simulink model "cantp"  (R2020a)
settings: Solver=VariableStepAuto  StartTime=0.0  StopTime=inf  RelTol=1e-3
InitFcn:
  | messagePeriod=1.0;%must be greater than 5ms.
  | 
  | Fsquare=1;
  | squareTs=0.01/Fsquare;
  | squareSamplesPerPeriod=fix(1/Fsquare/squareTs);
  | squareSamplesPerPulseWidth=fix(squareSamplesPerPeriod/2);
  | squareAmplitude=1;
  | 
  | Fsinus=0.05;
  | sinusTs=0.01/Fsinus;
  | sinusSamplesPerPeriod=fix(1/Fsinus/sinusTs);
  | sinusAmplitude=100;
  | rxCANSampleTime=0.01;
undefined symbols (not defined in the file): canChannel
libraries: canlib x14, canmsglib x14, simulink x6
(part 1 of 2)
settings Model: Creator=pc  LastModifiedBy=HP
settings DataIOCC: ReturnWorkspaceOutputs=off
settings DebuggingCC: ArithmeticOperatorsInVariantConditions=warning
settings SFSimCC: SimUseLocalCustomCode=off  CustomCodeUndefinedFunction=UseInterfaceOnly
settings RTWCC: RTWUseLocalCustomCode=off

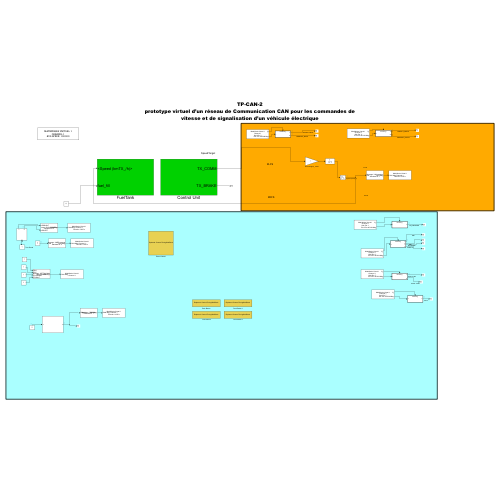
[thumbnail: Simulink's stored preview of the top-level diagram]
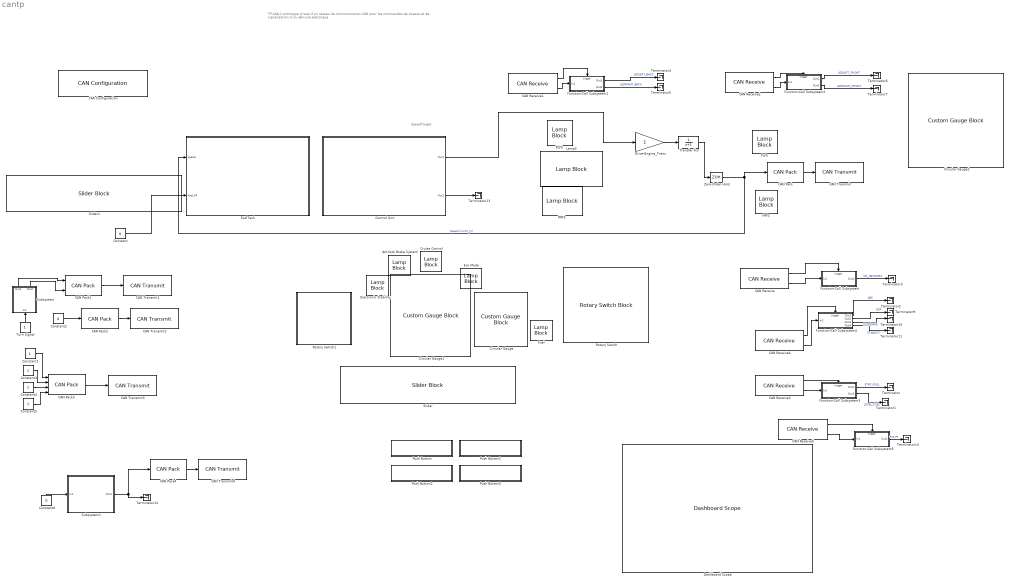
== system cantp ==
  note: SpeedTarget
  note: TP-CAN-2
      | prototype virtuel d’un réseau de Communication CAN pour les commandes de vitesse et de signalisation d’un véhicule électrique
  Antilock Brake System : LampBlock  LabelPosition=Hide  Icon=AntilockBrakeSystem
  CAN Configuration : canlib/CAN Configuration  BlockHandle=303.0002  Device=MathWorks Virtual 1 (Channel 1)  DeviceMenu=MathWorks Virtual 1 (Channel 1)  ObjConstructor=canChannel('MathWorks', 'Virtual 1', 1)  BusSpeed=100000  EnableBitParameters=off  AckMode=Normal
      settings: SourceProductBaseCode=VN
  CAN Pack : canmsglib/CAN Pack  MsgList=(none)  MsgName=VM message  MsgIDType=Standard (11-bit identifier)  MsgIdentifier=1  MsgLength=4  Remote=off  ApplyMinMax=off  BusOutput=off  SignalInfo={ 'VW', '0', '8', 'LE', 'unsigned', 'Standard', '0', '1', '0', '-Inf', 'Inf' }
      settings: SourceProductBaseCode=ME,XP,VN  DataFormat=manually specified signals
  CAN Pack1 : canmsglib/CAN Pack  MsgList=(none)  MsgName=DASHBOARD msg  MsgIDType=Standard (11-bit identifier)  MsgIdentifier=2  MsgLength=1  Remote=off  ApplyMinMax=off  BusOutput=off  SignalInfo={ 'LEDRIGHT', '0', '1', 'LE', 'unsigned', 'Standard', '0', '1', '0', '0', '1'; 'LEDLEFT', '1', '1', 'LE', 'unsigned', 'Standard', '0', '1', '0', '0', '1' }
      settings: SourceProductBaseCode=ME,XP,VN  DataFormat=manually specified signals
  CAN Pack2 : canmsglib/CAN Pack  MsgList=(none)  MsgName=VMES message  MsgIDType=Standard (11-bit identifier)  MsgIdentifier=3  MsgLength=2  Remote=off  ApplyMinMax=off  BusOutput=off  SignalInfo={ 'VM', '0', '8', 'LE', 'unsigned', 'Standard', '0', '1', '0', '0', '255' }
      settings: SourceProductBaseCode=ME,XP,VN  DataFormat=manually specified signals
  CAN Pack3 : canmsglib/CAN Pack  MsgList=(none)  MsgName=SETTING Msg  MsgIDType=Standard (11-bit identifier)  MsgIdentifier=6  MsgLength=1  Remote=off  ApplyMinMax=off  BusOutput=off  SignalInfo={ 'ABS', '0', '1', 'LE', 'unsigned', 'Standard', '0', '1', '0', '0', '1'; 'ESP', '1', '1', 'LE', 'unsigned', 'Standard', '0', '1', '0', '0', '1'; 'ECONOMIC', '2', '1', 'LE', 'unsigned', 'Standard', '0', '1', '0', '0', '1'; 'STABILIT', '3', '1', 'LE', 'unsigned', 'Standard', '0', '1', '0', '0', '1' }
      settings: SourceProductBaseCode=ME,XP,VN  DataFormat=manually specified signals
  CAN Pack4 : canmsglib/CAN Pack  MsgList=(none)  MsgName=CAN Msg  MsgIDType=Standard (11-bit identifier)  MsgIdentifier=7  MsgLength=1  Remote=off  ApplyMinMax=off  BusOutput=off  SignalInfo={ 'Signal1', '0', '1', 'LE', 'unsigned', 'Standard', '0', '1', '0', '0', '1' }
      settings: SourceProductBaseCode=ME,XP,VN  DataFormat=manually specified signals
  CAN Receive : canlib/CAN Receive  BlockHandle=309.0002  Device=MathWorks Virtual 1 (Channel 1)  DeviceMenu=MathWorks Virtual 1 (Channel 1)  ObjConstructor=canChannel('MathWorks', 'Virtual 1', 1)  EnableStandardIDsFilter=off  StdIDsCombo=Allow only  StandardIDs=1  EnableExtendedIDsFilter=off  ExtIDsCombo=Allow all  ExtendedIDs=0  SampleTime=0.01  MsgsPerTimestep=all  InternalFilterUpdateStatus=on  BusOutput=off
      settings: SourceProductBaseCode=VN
  CAN Receive1 : canlib/CAN Receive  BlockHandle=310.0002  Device=MathWorks Virtual 1 (Channel 1)  DeviceMenu=MathWorks Virtual 1 (Channel 1)  ObjConstructor=canChannel('MathWorks', 'Virtual 1', 1)  EnableStandardIDsFilter=off  StdIDsCombo=Allow only  StandardIDs=2  EnableExtendedIDsFilter=off  ExtIDsCombo=Allow all  ExtendedIDs=0  SampleTime=0.01  MsgsPerTimestep=all  InternalFilterUpdateStatus=on  BusOutput=off
      settings: SourceProductBaseCode=VN
  CAN Receive2 : canlib/CAN Receive  BlockHandle=528.0004  Device=MathWorks Virtual 1 (Channel 1)  DeviceMenu=MathWorks Virtual 1 (Channel 1)  ObjConstructor=canChannel('MathWorks', 'Virtual 1', 1)  EnableStandardIDsFilter=off  StdIDsCombo=Allow only  StandardIDs=2  EnableExtendedIDsFilter=off  ExtIDsCombo=Allow all  ExtendedIDs=0  SampleTime=0.01  MsgsPerTimestep=all  InternalFilterUpdateStatus=on  BusOutput=off
      settings: SourceProductBaseCode=VN
  CAN Receive3 : canlib/CAN Receive  BlockHandle=529.0004  Device=MathWorks Virtual 1 (Channel 1)  DeviceMenu=MathWorks Virtual 1 (Channel 1)  ObjConstructor=canChannel('MathWorks', 'Virtual 1', 1)  EnableStandardIDsFilter=off  StdIDsCombo=Allow only  StandardIDs=5  EnableExtendedIDsFilter=off  ExtIDsCombo=Allow all  ExtendedIDs=0  SampleTime=0.01  MsgsPerTimestep=all  InternalFilterUpdateStatus=on  BusOutput=off
      settings: SourceProductBaseCode=VN
  CAN Receive4 : canlib/CAN Receive  BlockHandle=530.0004  Device=MathWorks Virtual 1 (Channel 1)  DeviceMenu=MathWorks Virtual 1 (Channel 1)  ObjConstructor=canChannel('MathWorks', 'Virtual 1', 1)  EnableStandardIDsFilter=off  StdIDsCombo=Allow only  StandardIDs=6  EnableExtendedIDsFilter=off  ExtIDsCombo=Allow all  ExtendedIDs=0  SampleTime=0.01  MsgsPerTimestep=all  InternalFilterUpdateStatus=on  BusOutput=off
      settings: SourceProductBaseCode=VN
  CAN Receive5 : canlib/CAN Receive  BlockHandle=531.0002  Device=MathWorks Virtual 1 (Channel 1)  DeviceMenu=MathWorks Virtual 1 (Channel 1)  ObjConstructor=canChannel('MathWorks', 'Virtual 1', 1)  EnableStandardIDsFilter=off  StdIDsCombo=Allow only  StandardIDs=7  EnableExtendedIDsFilter=off  ExtIDsCombo=Allow all  ExtendedIDs=0  SampleTime=0.01  MsgsPerTimestep=all  InternalFilterUpdateStatus=on  BusOutput=off
      settings: SourceProductBaseCode=VN
  CAN Transmit : canlib/CAN Transmit  BlockHandle=532.0002  Device=MathWorks Virtual 1 (Channel 1)  DeviceMenu=MathWorks Virtual 1 (Channel 1)  ObjConstructor=canChannel('MathWorks', 'Virtual 1', 1)  EnableEventTransmit=off  EnablePeriodicTransmit=on  MessagePeriod=0.025
      settings: SourceProductBaseCode=VN
  CAN Transmit1 : canlib/CAN Transmit  BlockHandle=533.0002  Device=MathWorks Virtual 1 (Channel 1)  DeviceMenu=MathWorks Virtual 1 (Channel 1)  ObjConstructor=canChannel('MathWorks', 'Virtual 1', 1)  EnableEventTransmit=off  EnablePeriodicTransmit=on  MessagePeriod=0.025
      settings: SourceProductBaseCode=VN
  CAN Transmit2 : canlib/CAN Transmit  BlockHandle=534.0002  Device=MathWorks Virtual 1 (Channel 1)  DeviceMenu=MathWorks Virtual 1 (Channel 1)  ObjConstructor=canChannel('MathWorks', 'Virtual 1', 1)  EnableEventTransmit=off  EnablePeriodicTransmit=on  MessagePeriod=0.025
      settings: SourceProductBaseCode=VN
  CAN Transmit3 : canlib/CAN Transmit  BlockHandle=535.0002  Device=MathWorks Virtual 1 (Channel 1)  DeviceMenu=MathWorks Virtual 1 (Channel 1)  ObjConstructor=canChannel('MathWorks', 'Virtual 1', 1)  EnableEventTransmit=off  EnablePeriodicTransmit=off  MessagePeriod=1.000
      settings: SourceProductBaseCode=VN
  CAN Transmit4 : canlib/CAN Transmit  BlockHandle=536.0002  Device=MathWorks Virtual 1 (Channel 1)  DeviceMenu=MathWorks Virtual 1 (Channel 1)  ObjConstructor=canChannel('MathWorks', 'Virtual 1', 1)  EnableEventTransmit=off  EnablePeriodicTransmit=on  MessagePeriod=0.025
      settings: SourceProductBaseCode=VN
  Circular Gauge : CustomGaugeBlock  LabelPosition=Hide  ShowInitialText=on  LabelPosition=Hide  ScaleMin=0  ScaleMax=100  TickInterval=auto  fixedAspectRatio=on  GaugeMin=0  GaugeMax=100  GaugeArcDefined=true  GaugeArcRadius=0.18125  GaugeArcStrokeWidth=0.03295454545454546  GaugeArcColor=#fcfcc5  GaugeArcRotation=225  GaugeArcRatio=0.75  GaugeArcTransparency=0  ValueArcTransparency=1  ValueArcColor=#0072bd  GaugeTickVisible=1  GaugeTickTransparency=1  GaugeTickColor=#fcfcc5  ScaleColorsJSON=[]  CenterOffsetX=-0.00375  CenterOffsetY=-0.00515625  NeedleImage=data:image/svg+xml;base64,PD94bWwgdmVyc2lvbj0iMS4wIiBlbmNvZGluZz0idXRmLTgiPz4KPCEtLSBHZW5lcmF0b3I6IEFkb2JlIElsbHVzdHJhdG9yIDI0LjEuMiwgU1ZHIEV4cG9ydCBQbHVnLUluIC4gU1ZHIFZlcnNpb246IDYuMDAgQnVpbGQgMCkgIC0tPgo8c3ZnIHZlcnNpb249IjEuMSIgaWQ9IkxheWVyXzEiIHhtbG5zPSJodHRwOi8vd3d3LnczLm9yZy8yMDAwL3N2ZyIgeG1sbnM6eGxpbms9Imh0dHA6Ly93d3cudzMub3JnLzE5OTkveGxpbmsiIHg9IjBweCIgeT0iMHB4IgoJIHZpZXdCb3g9IjAgMCAyMDAgNTAiIHN0eWxlPSJlbmFibGUtYmFja2dyb3VuZDpuZXcgMCAwIDIwMCA1MDsiIHhtbDpzcGFjZT0icHJlc2VydmUiPgo8c3R5bGUgdHlwZT0idGV4dC9jc3MiPgoJLnN0MHtmaWxsOiNFQzIxMjc7fQo8L3N0eWxlPgo8cGF0aCBjbGFzcz0ic3QwIiBkPSJNMTYyLjgsMTMuN0MxNjksNC40LDE4MS43LDEuOSwxOTEsOC4xczExLjgsMTguOSw1LjYsMjguMnMtMTguOSwxMS44LTI4LjIsNS42bDAsMAoJQzE1OS4xLDM1LjYsMTU2LjYsMjMsMTYyLjgsMTMuN0wxNjIuOCwxMy43eiBNMTY1LjgsMTUuOGMtNS4xLDcuNi0zLjEsMTcuOSw0LjYsMjNjNy42LDUuMSwxNy45LDMuMSwyMy00LjYKCWM1LjEtNy42LDMuMS0xNy45LTQuNi0yM2wwLDBDMTgxLjIsNi4yLDE3MC45LDguMiwxNjUuOCwxNS44eiIvPgo8cGF0aCBjbGFzcz0ic3QwIiBkPSJNMC40LDI1Ljl2LTMuM2wxNTktMi41Yy0wLjcsMi42LTAuNyw1LjIsMCw3LjhMMC40LDI1Ljl6Ii8+CjxjaXJjbGUgY2xhc3M9InN0MCIgY3g9IjE3OS42IiBjeT0iMjQiIHI9IjAuNyIvPgo8L3N2Zz4K  NeedleXPos=0.3459906005859375  NeedleYPos=0.5370294189453125  NeedleHeight=0.05870846152673457  NeedleWidth=0.23054168772545627  NeedleInitialRotation=-45  BackgroundImage=data:image/svg+xml;base64,PD94bWwgdmVyc2lvbj0iMS4wIiBlbmNvZGluZz0iVVRGLTgiIHN0YW5kYWxvbmU9Im5vIj8+CjxzdmcKICAgeG1sbnM6ZGM9Imh0dHA6Ly9wdXJsLm9yZy9kYy9lbGVtZW50cy8xLjEvIgogICB4bWxuczpjYz0iaHR0cDovL2NyZWF0aXZlY29tbW9ucy5vcmcvbnMjIgogICB4bWxuczpyZGY9Imh0dHA6Ly93d3cudzMub3JnLzE5OTkvMDIvMjItcmRmLXN5bnRheC1ucyMiCiAgIHhtbG5zOnN2Zz0iaHR0cDovL3d3dy53My5vcmcvMjAwMC9zdmciCiAgIHhtbG5zPSJodHRwOi8vd3d3LnczLm9yZy8yMDAwL3N2ZyIKICAgeG1sbnM6 ...(+9964 chars)
  Circular Gauge1 : CustomGaugeBlock  LabelPosition=Hide  ShowInitialText=on  LabelPosition=Hide  ScaleMin=0  ScaleMax=240  TickInterval=auto  fixedAspectRatio=on  GaugeMin=0  GaugeMax=240  GaugeArcDefined=true  GaugeArcRadius=0.18032212885154061  GaugeArcStrokeWidth=0.03278584160937103  GaugeArcColor=#fcfcc5  GaugeArcRotation=225  GaugeArcRatio=0.75  GaugeArcTransparency=0  ValueArcTransparency=1  ValueArcColor=#0072bd  GaugeTickVisible=1  GaugeTickTransparency=1  GaugeTickColor=#fcfcc5  ScaleColorsJSON=[]  CenterOffsetX=-0.00375  CenterOffsetY=0.0027573529411764708  NeedleImage=data:image/svg+xml;base64,PD94bWwgdmVyc2lvbj0iMS4wIiBlbmNvZGluZz0idXRmLTgiPz4KPCEtLSBHZW5lcmF0b3I6IEFkb2JlIElsbHVzdHJhdG9yIDI0LjEuMiwgU1ZHIEV4cG9ydCBQbHVnLUluIC4gU1ZHIFZlcnNpb246IDYuMDAgQnVpbGQgMCkgIC0tPgo8c3ZnIHZlcnNpb249IjEuMSIgaWQ9IkxheWVyXzEiIHhtbG5zPSJodHRwOi8vd3d3LnczLm9yZy8yMDAwL3N2ZyIgeG1sbnM6eGxpbms9Imh0dHA6Ly93d3cudzMub3JnLzE5OTkveGxpbmsiIHg9IjBweCIgeT0iMHB4IgoJIHZpZXdCb3g9IjAgMCAyMDAgNTAiIHN0eWxlPSJlbmFibGUtYmFja2dyb3VuZDpuZXcgMCAwIDIwMCA1MDsiIHhtbDpzcGFjZT0icHJlc2VydmUiPgo8c3R5bGUgdHlwZT0idGV4dC9jc3MiPgoJLnN0MHtmaWxsOiNFQzIxMjc7fQo8L3N0eWxlPgo8cGF0aCBjbGFzcz0ic3QwIiBkPSJNMTYyLjgsMTMuN0MxNjksNC40LDE4MS43LDEuOSwxOTEsOC4xczExLjgsMTguOSw1LjYsMjguMnMtMTguOSwxMS44LTI4LjIsNS42bDAsMAoJQzE1OS4xLDM1LjYsMTU2LjYsMjMsMTYyLjgsMTMuN0wxNjIuOCwxMy43eiBNMTY1LjgsMTUuOGMtNS4xLDcuNi0zLjEsMTcuOSw0LjYsMjNjNy42LDUuMSwxNy45LDMuMSwyMy00LjYKCWM1LjEtNy42LDMuMS0xNy45LTQuNi0yM2wwLDBDMTgxLjIsNi4yLDE3MC45LDguMiwxNjUuOCwxNS44eiIvPgo8cGF0aCBjbGFzcz0ic3QwIiBkPSJNMC40LDI1Ljl2LTMuM2wxNTktMi41Yy0wLjcsMi42LTAuNyw1LjIsMCw3LjhMMC40LDI1Ljl6Ii8+CjxjaXJjbGUgY2xhc3M9InN0MCIgY3g9IjE3OS42IiBjeT0iMjQiIHI9IjAuNyIvPgo8L3N2Zz4K  NeedleXPos=0.34361348470052083  NeedleYPos=0.5332382301879085  NeedleHeight=0.05870846152673456  NeedleWidth=0.2260212624759375  NeedleInitialRotation=-45  BackgroundImage=data:image/svg+xml;base64,PD94bWwgdmVyc2lvbj0iMS4wIiBlbmNvZGluZz0iVVRGLTgiIHN0YW5kYWxvbmU9Im5vIj8+CjxzdmcKICAgeG1sbnM6ZGM9Imh0dHA6Ly9wdXJsLm9yZy9kYy9lbGVtZW50cy8xLjEvIgogICB4bWxuczpjYz0iaHR0cDovL2NyZWF0aXZlY29tbW9ucy5vcmcvbnMjIgogICB4bWxuczpyZGY9Imh0dHA6Ly93d3cudzMub3JnLzE5OTkvMDIvMjItcmRmLXN5bnRheC1ucyMiCiAgIHhtbG5zOnN2Zz0iaHR0cDovL3d3dy53My5vcmcvMjAwMC9zdmciCiAgIHhtbG5zPSJodHRwOi8vd3d3LnczLm9yZy8yMDAwL3N2ZyIKICAgeG1sbnM6 ...(+9964 chars)
  Circular Gauge2 : CustomGaugeBlock  LabelPosition=Hide  ShowInitialText=on  LabelPosition=Hide  ScaleMin=0  ScaleMax=1  TickInterval=auto  fixedAspectRatio=on  GaugeMin=0  GaugeMax=1  GaugeArcDefined=true  GaugeArcRadius=0.1781875438904494  GaugeArcStrokeWidth=0.03239773525280899  GaugeArcColor=#fcfcc5  GaugeArcRotation=225  GaugeArcRatio=0.75  GaugeArcTransparency=0  ValueArcTransparency=0  ValueArcColor=#0072bd  GaugeTickVisible=1  GaugeTickTransparency=0  GaugeTickColor=#fcfcc5  ScaleColorsJSON=[]  CenterOffsetX=0.00008778089887640449  CenterOffsetY=-0.0009821428571428572  NeedleImage=data:image/svg+xml;base64,PD94bWwgdmVyc2lvbj0iMS4wIiBlbmNvZGluZz0idXRmLTgiPz4KPCEtLSBHZW5lcmF0b3I6IEFkb2JlIElsbHVzdHJhdG9yIDI0LjEuMiwgU1ZHIEV4cG9ydCBQbHVnLUluIC4gU1ZHIFZlcnNpb246IDYuMDAgQnVpbGQgMCkgIC0tPgo8c3ZnIHZlcnNpb249IjEuMSIgaWQ9IkxheWVyXzEiIHhtbG5zPSJodHRwOi8vd3d3LnczLm9yZy8yMDAwL3N2ZyIgeG1sbnM6eGxpbms9Imh0dHA6Ly93d3cudzMub3JnLzE5OTkveGxpbmsiIHg9IjBweCIgeT0iMHB4IgoJIHZpZXdCb3g9IjAgMCAyMDAgNTAiIHN0eWxlPSJlbmFibGUtYmFja2dyb3VuZDpuZXcgMCAwIDIwMCA1MDsiIHhtbDpzcGFjZT0icHJlc2VydmUiPgo8c3R5bGUgdHlwZT0idGV4dC9jc3MiPgoJLnN0MHtmaWxsOiNFQzIxMjc7fQo8L3N0eWxlPgo8cGF0aCBjbGFzcz0ic3QwIiBkPSJNMTYyLjgsMTMuN0MxNjksNC40LDE4MS43LDEuOSwxOTEsOC4xczExLjgsMTguOSw1LjYsMjguMnMtMTguOSwxMS44LTI4LjIsNS42bDAsMAoJQzE1OS4xLDM1LjYsMTU2LjYsMjMsMTYyLjgsMTMuN0wxNjIuOCwxMy43eiBNMTY1LjgsMTUuOGMtNS4xLDcuNi0zLjEsMTcuOSw0LjYsMjNjNy42LDUuMSwxNy45LDMuMSwyMy00LjYKCWM1LjEtNy42LDMuMS0xNy45LTQuNi0yM2wwLDBDMTgxLjIsNi4yLDE3MC45LDguMiwxNjUuOCwxNS44eiIvPgo8cGF0aCBjbGFzcz0ic3QwIiBkPSJNMC40LDI1Ljl2LTMuM2wxNTktMi41Yy0wLjcsMi42LTAuNyw1LjIsMCw3LjhMMC40LDI1Ljl6Ii8+CjxjaXJjbGUgY2xhc3M9InN0MCIgY3g9IjE3OS42IiBjeT0iMjQiIHI9IjAuNyIvPgo8L3N2Zz4K  NeedleXPos=0.45904198121488765  NeedleYPos=0.5336383492606026  NeedleHeight=0.0577189930740368  NeedleWidth=0.23054168772545627  NeedleInitialRotation=-45  BackgroundImage=data:image/svg+xml;base64,PD94bWwgdmVyc2lvbj0iMS4wIiBlbmNvZGluZz0iVVRGLTgiIHN0YW5kYWxvbmU9Im5vIj8+CjxzdmcKICAgeG1sbnM6ZGM9Imh0dHA6Ly9wdXJsLm9yZy9kYy9lbGVtZW50cy8xLjEvIgogICB4bWxuczpjYz0iaHR0cDovL2NyZWF0aXZlY29tbW9ucy5vcmcvbnMjIgogICB4bWxuczpyZGY9Imh0dHA6Ly93d3cudzMub3JnLzE5OTkvMDIvMjItcmRmLXN5bnRheC1ucyMiCiAgIHhtbG5zOnN2Zz0iaHR0cDovL3d3dy53My5vcmcvMjAwMC9zdmciCiAgIHhtbG5zPSJodHRwOi8vd3d3LnczLm9yZy8yMDAwL3N2ZyIKICAgeG1sbnM6 ...(+9964 chars)
  Constant : Constant  Value=0
  Constant{1,3..5} (4 alike) : Constant  SampleTime=0.01
  Constant2 : Constant  Value=0  OutMin=0  OutMax=240  SampleTime=0.001
  Constant6 : Constant  Value=0
  Control Unit : Subsystem
  Cruise Control : LampBlock  LabelPosition=Hide  Icon=CruiseControl
  Dashboard Scope : DashboardScope  Ymin=-50  Ymax=250
  Drive-Engine_Trans : Gain
  Eco Mode : LampBlock  LabelPosition=Hide  Icon=EcoMode
  Electronic Stability : LampBlock  LabelPosition=Hide  Icon=ElectronicStability
  FLFS : LampBlock
  FRFS : LampBlock
  Fuel : LampBlock  LabelPosition=Hide  Icon=Fuel
  FuelTank : Subsystem
  Function-Call Subsystem : Subsystem  TreatAsAtomicUnit=on
  Function-Call Subsystem1 : Subsystem  TreatAsAtomicUnit=on
  Function-Call Subsystem2 : Subsystem  TreatAsAtomicUnit=on
  Function-Call Subsystem3 : Subsystem  TreatAsAtomicUnit=on
  Function-Call Subsystem4 : Subsystem  TreatAsAtomicUnit=on
  Function-Call Subsystem5 : Subsystem  TreatAsAtomicUnit=on
  Lamp3 : LampBlock
  Push Button : Subsystem  Description=Replaced Block  mask(Replaced Block){}
      mask help: This block has been replaced with an empty subsystem because it used functionality that is unavailable in Simulink R2020a.
      mask Display: fprintf('Replaced: %s\n','CustomTuningWebBlock')
  Push Button1 : Subsystem  Description=Replaced Block  mask(Replaced Block){}
      mask help: This block has been replaced with an empty subsystem because it used functionality that is unavailable in Simulink R2020a.
      mask Display: fprintf('Replaced: %s\n','CustomTuningWebBlock')
  Push Button2 : Subsystem  Description=Replaced Block  mask(Replaced Block){}
      mask help: This block has been replaced with an empty subsystem because it used functionality that is unavailable in Simulink R2020a.
      mask Display: fprintf('Replaced: %s\n','CustomTuningWebBlock')
  Push Button3 : Subsystem  Description=Replaced Block  mask(Replaced Block){}
      mask help: This block has been replaced with an empty subsystem because it used functionality that is unavailable in Simulink R2020a.
      mask Display: fprintf('Replaced: %s\n','CustomTuningWebBlock')
  RLFS : LampBlock
  RRFS : LampBlock
  Rotary Switch : RotarySwitchBlock
      settings: Values={{'Off', 'Low', 'Medium', 'High'}, [0 1 2 3]}
  Rotary Switch1 : Subsystem  Description=Replaced Block  mask(Replaced Block){}
      mask help: This block has been replaced with an empty subsystem because it used functionality that is unavailable in Simulink R2020a.
      mask Display: fprintf('Replaced: %s\n','CustomTuningWebBlock')
  Slider : SliderBlock  ScaleMax=240
  Slider1 : SliderBlock
  Subsystem : Subsystem
  Subsystem1 : Subsystem
  Terminator{,1..7,9..14} (14 alike) : Terminator
  Transfer Fcn : TransferFcn  Numerator=1  Denominator=[ 1 1]
  "Turn Signal " : Constant  OutMin=0  OutMax=240
  Zero-Order Hold : ZeroOrderHold  SampleTime=0.01
  wires:
  Drive-Engine_Trans/1 -> Transfer Fcn/1
  Transfer Fcn/1 -> Zero-Order Hold/1
  Zero-Order Hold/1 -> FuelTank/1(speed), CAN Pack/1  "Speed (kmTX_/h)"
  "Turn Signal "/1 -> Subsystem/1(In1)
  Subsystem/2(Out2) -> CAN Pack1/2
  CAN Pack/1 -> CAN Transmit/1
  CAN Receive/2 -> Function-Call Subsystem/1(In1)
  CAN Receive/1 -> Function-Call Subsystem/Trigger
  Function-Call Subsystem/1(Out1) -> Terminator3/1  "VM_NETWORK"
  CAN Pack1/1 -> CAN Transmit1/1
  Subsystem/1(Out1) -> CAN Pack1/1
  CAN Receive1/2 -> Function-Call Subsystem1/1(In1)
  CAN Receive1/1 -> Function-Call Subsystem1/Trigger
  Function-Call Subsystem1/1(Out1) -> Terminator4/1  "LEDLEFT_BACK"
  Function-Call Subsystem1/2(Out2) -> Terminator5/1  "LEDRIGHT_BACK"
  CAN Receive2/2 -> Function-Call Subsystem2/1(In1)
  CAN Receive2/1 -> Function-Call Subsystem2/Trigger
  Function-Call Subsystem2/2(Out2) -> Terminator7/1  "LEDRIGHT_FRONT"
  Function-Call Subsystem2/1(Out1) -> Terminator6/1  "LEDLEFT_FRONT"
  CAN Pack2/1 -> CAN Transmit2/1
  Constant2/1 -> CAN Pack2/1
  Constant/1 -> FuelTank/2(fuel_fill)
  CAN Receive3/2 -> Function-Call Subsystem3/1(In1)
  CAN Receive3/1 -> Function-Call Subsystem3/Trigger
  Function-Call Subsystem3/1(Out1) -> Terminator/1  "ETAT_FUEL"
  Function-Call Subsystem3/2(Out2) -> Terminator1/1  "LEVEL_FUEL"
  CAN Pack3/1 -> CAN Transmit3/1
  CAN Receive4/1 -> Function-Call Subsystem4/Trigger
  CAN Receive4/2 -> Function-Call Subsystem4/1(In1)
  Constant1/1 -> CAN Pack3/1
  Constant3/1 -> CAN Pack3/2
  Constant4/1 -> CAN Pack3/3
  Constant5/1 -> CAN Pack3/4
  Function-Call Subsystem4/1(Out1) -> Terminator2/1  "ABS"
  Function-Call Subsystem4/2(Out2) -> Terminator9/1  "ESP"
  Function-Call Subsystem4/3(Out3) -> Terminator10/1  "ECONOMIE"
  Function-Call Subsystem4/4(Out4) -> Terminator11/1  "STABILITY"
  Subsystem1/1(Out1) -> CAN Pack4/1, Terminator12/1
  Control Unit/1(Out1) -> Drive-Engine_Trans/1
  Control Unit/2(Out2) -> Terminator13/1
  Constant6/1 -> Subsystem1/1(In1)
  CAN Pack4/1 -> CAN Transmit4/1
  CAN Receive5/2 -> Function-Call Subsystem5/1(In1)
  CAN Receive5/1 -> Function-Call Subsystem5/Trigger
  Function-Call Subsystem5/1(Out1) -> Terminator14/1  "essuie"
